simulink model "LEO_SATCOM_BeamSteering"  (R2025b)
settings: Solver=ode3  StartTime=0.0  StopTime=1e-4  FixedStep=5e-08  RelTol=1e-3
settings Model: Creator=AYAN DAS  LastModifiedBy=AYAN DAS

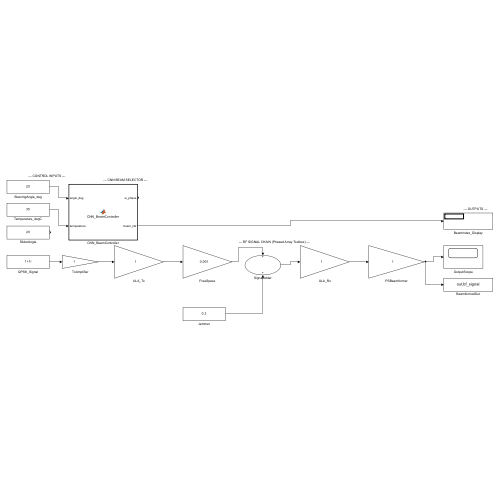
[thumbnail: Simulink's stored preview of the top-level diagram]
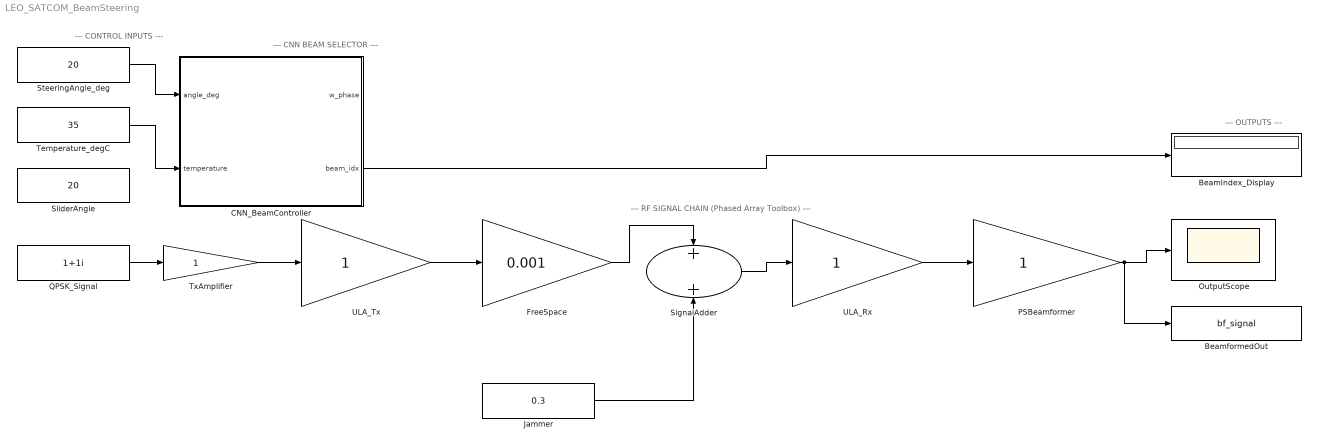
== system LEO_SATCOM_BeamSteering ==
  note: --- CONTROL INPUTS ---
  note: --- CNN BEAM SELECTOR ---
  note: --- RF SIGNAL CHAIN (Phased Array Toolbox) ---
  note: --- OUTPUTS ---
  BeamIndex_Display : Display
  BeamformedOut : ToWorkspace  VariableName=bf_signal  SampleTime=-1
  CNN_BeamController : MATLAB Function  TreatAsAtomicUnit=on
  FreeSpace : Gain  Gain=0.001
  Jammer : Constant  Value=0.3  OutDataTypeStr=double
  OutputScope : Scope
  PSBeamformer : Gain
  QPSK_Signal : Constant  Value=1+1i  OutDataTypeStr=double
  SignalAdder : Sum
  SliderAngle : Constant  Value=20  OutDataTypeStr=double
  SteeringAngle_deg : Constant  Value=20  VectorParams1D=off  OutDataTypeStr=double
  Temperature_degC : Constant  Value=35  VectorParams1D=off  OutDataTypeStr=double
  TxAmplifier : Gain
  ULA_Rx : Gain
  ULA_Tx : Gain
  wires:
  SteeringAngle_deg/1 -> CNN_BeamController/1(angle_deg)
  Temperature_degC/1 -> CNN_BeamController/2(temperature)
  CNN_BeamController/2(beam_idx) -> BeamIndex_Display/1
  QPSK_Signal/1 -> TxAmplifier/1
  TxAmplifier/1 -> ULA_Tx/1
  ULA_Tx/1 -> FreeSpace/1
  FreeSpace/1 -> SignalAdder/1
  Jammer/1 -> SignalAdder/2
  SignalAdder/1 -> ULA_Rx/1
  ULA_Rx/1 -> PSBeamformer/1
  PSBeamformer/1 -> OutputScope/1, BeamformedOut/1

== matlab function LEO_SATCOM_BeamSteering/CNN_BeamController ==
  data: angle_deg input; w_phase output; temperature input; beam_idx output
function [w_phase, beam_idx] = CNN_BeamController(angle_deg, temperature)
